simulink model "simulink_app"  (R2015a)
settings: Solver=ode2  SolverMode=SingleTasking  StartTime=0.0  StopTime=inf  FixedStep=T_ctrl  RelTol=1e-3
undefined symbols (not defined in the file): A_l_max_x, A_l_max_y, A_z_max, B_hover_4dof, CG_0, epsilon, eta_23, g, h, h_M, Hover_eta_23, Hover_throtle_1, Hover_throtle_23, I_BAC_0, Ix, Iy, Iz, l, l_arm, m, m_0, m_M, Rotation_sign, T_ctrl, throtle_1, throtle_23, v_i0
libraries: XXCopter_Control x52, simulink x11, XXCopter x1
(part 3 of 4)

== system simulink_app/Flight mode manager and commands generator/Commands generator/Take off ==
  Init comands : Inport
  Gains : Inport  Port=2
  Left_up : Inport  Port=3
  Left_side : Inport  Port=4
  Right_up : Inport  Port=5
  Right_side : Inport  Port=6
  GCS_comm : Inport  Port=7
  Enable : EnablePort  StatesWhenEnabling=reset  ShowOutputPort=on
  Bus Selector : BusSelector  OutputSignals=K_alt
  Bus Selector1 : BusSelector  OutputSignals=Alt_sp
  Bus Selector2 : BusSelector  OutputSignals=Alt_com
  Divide : Product  Inputs=**
  GCS params safemode : XXCopter_Control/GCS params safemode
  Ground{,1..4} (5 alike) : Ground
  Mux : Mux  Inputs=[2,1]
  Mux1 : Mux  Inputs=[2,1]
  Mux2 : Mux  Inputs=3
  Sum : Sum  Inputs=|++
  Sum1 : Sum  Inputs=|++
  Terminator : Terminator
  Terminator1 : Terminator
  Terminator2 : Terminator
  Unary Minus : UnaryMinus
  Pos_ref(m) : Outport
  Vel_ref_yaw(mps) : Outport  Port=2
  Att_ref(rad) : Outport  Port=3
  omega_b_ref : Outport  Port=4
  wires:
  Mux1/1 -> Vel_ref_yaw(mps)/1
  Mux/1 -> Pos_ref(m)/1
  Mux2/1 -> Att_ref(rad)/1
  Gains/1 -> Bus Selector/1
  Init comands/1 -> Bus Selector1/1
  Unary Minus/1 -> Mux/2
  GCS_comm/1 -> Bus Selector2/1
  Bus Selector1/1 -> Sum/1  "<Alt_sp>"
  Bus Selector/1 -> Divide/1  "<K_alt>"
  Left_up/1 -> Divide/2
  Divide/1 -> Sum/2
  Sum/1 -> Sum1/1
  GCS params safemode/1 -> Sum1/2
  Sum1/1 -> Unary Minus/1
  Right_up/1 -> Terminator/1
  Left_side/1 -> Terminator1/1
  Right_side/1 -> Terminator2/1
  Ground/1 -> omega_b_ref/1
  Ground1/1 -> Mux2/3, Mux2/2, Mux2/1
  Ground2/1 -> Mux1/1
  Ground3/1 -> Mux1/2
  Ground4/1 -> Mux/1
  Enable/1 -> GCS params safemode/1
  Bus Selector2/1 -> GCS params safemode/2  "<Alt_com>"

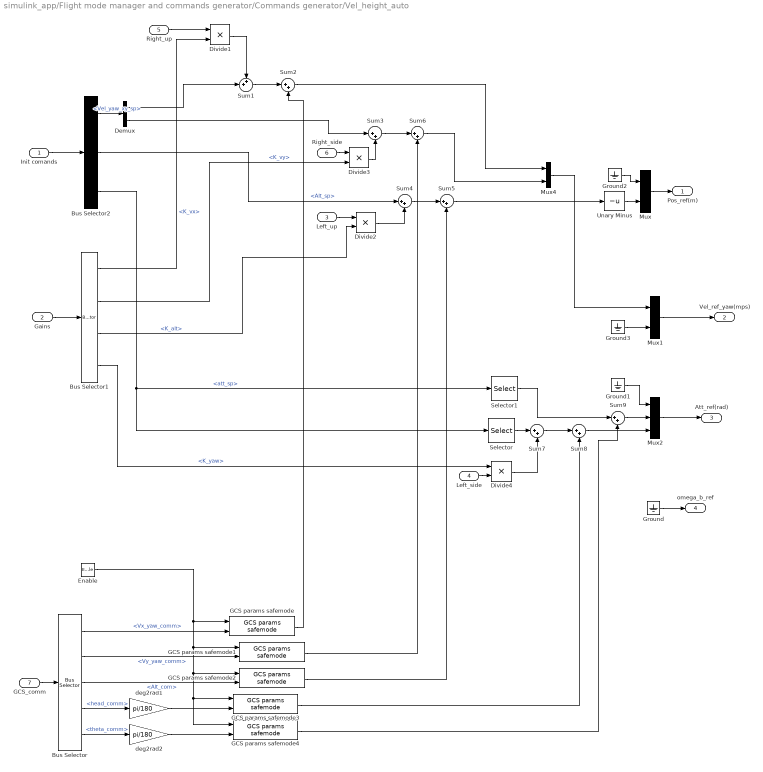
== system simulink_app/Flight mode manager and commands generator/Commands generator/Vel_height_auto ==
  Init comands : Inport
  Gains : Inport  Port=2
  Left_up : Inport  Port=3
  Left_side : Inport  Port=4
  Right_up : Inport  Port=5
  Right_side : Inport  Port=6
  GCS_comm : Inport  Port=7
  Enable : EnablePort  StatesWhenEnabling=reset  ShowOutputPort=on
  Bus Selector : BusSelector  OutputSignals=Vx_yaw_comm,Vy_yaw_comm,Alt_com,head_comm,theta_comm
  Bus Selector1 : BusSelector  OutputSignals=K_vx,K_vy,K_alt,K_yaw
  Bus Selector2 : BusSelector  OutputSignals=Vel_yaw_xy_sp,Alt_sp,att_sp
  Demux : Demux  Outputs=2
  Divide{1..4} (4 alike) : Product  Inputs=**
  GCS params safemode{,1..4} (5 alike) : XXCopter_Control/GCS params safemode
  Ground{,1..3} (4 alike) : Ground
  Mux : Mux  Inputs=[2,1]
  Mux1 : Mux  Inputs=[2,1]
  Mux2 : Mux  Inputs=3
  Mux4 : Mux  Inputs=2
  Selector : Selector  InputPortWidth=3  Indices=3
  Selector1 : Selector  InputPortWidth=3  Indices=2
  Sum1 : Sum  Inputs=++|
  Sum{2..9} (8 alike) : Sum  Inputs=|++
  Unary Minus : UnaryMinus
  deg2rad1 : Gain  Gain=pi/180
  deg2rad2 : Gain  Gain=pi/180
  Pos_ref(m) : Outport
  Vel_ref_yaw(mps) : Outport  Port=2
  Att_ref(rad) : Outport  Port=3
  omega_b_ref : Outport  Port=4
  wires:
  Mux1/1 -> Vel_ref_yaw(mps)/1
  Mux2/1 -> Att_ref(rad)/1
  Unary Minus/1 -> Mux/2
  Ground1/1 -> Mux2/1
  Mux4/1 -> Mux1/1
  Ground3/1 -> Mux1/2
  Ground/1 -> omega_b_ref/1
  Mux/1 -> Pos_ref(m)/1
  Gains/1 -> Bus Selector1/1
  Init comands/1 -> Bus Selector2/1
  GCS_comm/1 -> Bus Selector/1
  Sum4/1 -> Sum5/1
  Divide2/1 -> Sum4/2
  Bus Selector2/2 -> Sum4/1  "<Alt_sp>"
  Bus Selector2/1 -> Demux/1  "<Vel_yaw_xy_sp>"
  Sum1/1 -> Sum2/1
  Demux/1 -> Sum1/2
  Right_up/1 -> Divide1/1
  Divide1/1 -> Sum1/1
  Bus Selector1/1 -> Divide1/2  "<K_vx>"
  Bus Selector/1 -> GCS params safemode/2  "<Vx_yaw_comm>"
  GCS params safemode/1 -> Sum2/2
  Bus Selector/2 -> GCS params safemode1/2  "<Vy_yaw_comm>"
  Bus Selector/3 -> GCS params safemode2/2  "<Alt_com>"
  Bus Selector/4 -> deg2rad1/1  "<head_comm>"
  Bus Selector/5 -> deg2rad2/1  "<theta_comm>"
  GCS params safemode2/1 -> Sum5/2
  Sum5/1 -> Unary Minus/1
  Bus Selector1/3 -> Divide2/2  "<K_alt>"
  Left_up/1 -> Divide2/1
  Sum3/1 -> Sum6/1
  Divide3/1 -> Sum3/2
  Right_side/1 -> Divide3/1
  Bus Selector1/2 -> Divide3/2  "<K_vy>"
  Demux/2 -> Sum3/1
  Sum2/1 -> Mux4/1
  Sum6/1 -> Mux4/2
  GCS params safemode1/1 -> Sum6/2
  Sum7/1 -> Sum8/1
  Selector/1 -> Sum7/1
  Left_side/1 -> Divide4/2
  Bus Selector2/3 -> Selector/1, Selector1/1  "<att_sp>"
  Bus Selector1/4 -> Divide4/1  "<K_yaw>"
  Sum8/1 -> Mux2/3
  Selector1/1 -> Sum9/1
  Sum9/1 -> Mux2/2
  Divide4/1 -> Sum7/2
  GCS params safemode3/1 -> Sum8/2
  GCS params safemode4/1 -> Sum9/2
  Ground2/1 -> Mux/1
  deg2rad1/1 -> GCS params safemode3/2
  deg2rad2/1 -> GCS params safemode4/2
  Enable/1 -> GCS params safemode4/1, GCS params safemode3/1, GCS params safemode2/1, GCS params safemode1/1, GCS params safemode/1

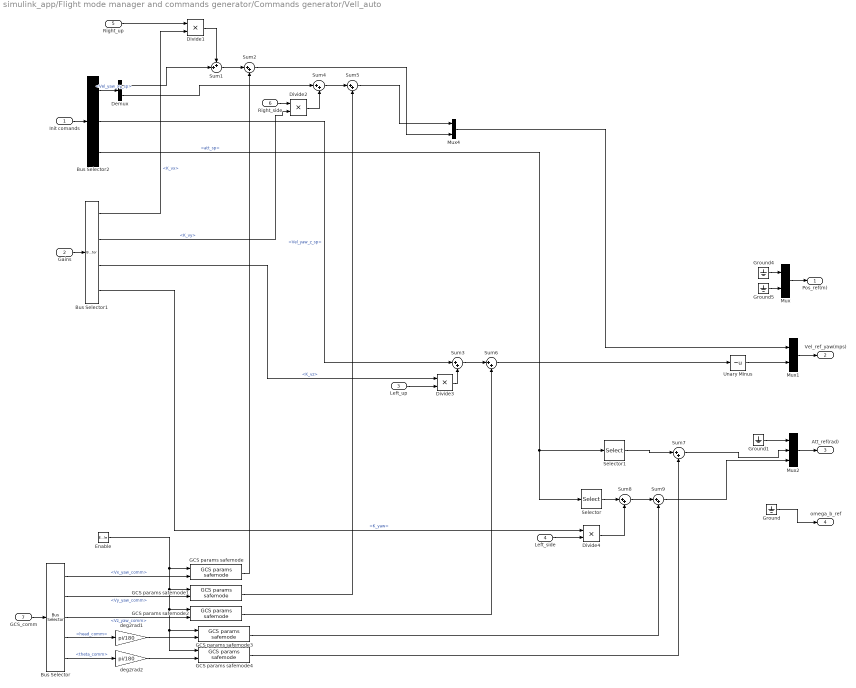
== system simulink_app/Flight mode manager and commands generator/Commands generator/Vell_auto ==
  Init comands : Inport
  Gains : Inport  Port=2
  Left_up : Inport  Port=3
  Left_side : Inport  Port=4
  Right_up : Inport  Port=5
  Right_side : Inport  Port=6
  GCS_comm : Inport  Port=7
  Enable : EnablePort  StatesWhenEnabling=reset  ShowOutputPort=on
  Bus Selector : BusSelector  OutputSignals=Vx_yaw_comm,Vy_yaw_comm,Vz_yaw_comm,head_comm,theta_comm
  Bus Selector1 : BusSelector  OutputSignals=K_vx,K_vy,K_vz,K_yaw
  Bus Selector2 : BusSelector  OutputSignals=Vel_yaw_xy_sp,Vel_yaw_z_sp,att_sp
  Demux : Demux  Outputs=2
  Divide{1..4} (4 alike) : Product  Inputs=**
  GCS params safemode{,1..4} (5 alike) : XXCopter_Control/GCS params safemode
  Ground{,1,4..5} (4 alike) : Ground
  Mux : Mux  Inputs=[2,1]
  Mux1 : Mux  Inputs=[2,1]
  Mux2 : Mux  Inputs=3
  Mux4 : Mux  Inputs=2
  Selector : Selector  InputPortWidth=3  Indices=3
  Selector1 : Selector  InputPortWidth=3  Indices=2
  Sum1 : Sum  Inputs=++|
  Sum{2..9} (8 alike) : Sum  Inputs=|++
  Unary Minus : UnaryMinus
  deg2rad1 : Gain  Gain=pi/180
  deg2rad2 : Gain  Gain=pi/180
  Pos_ref(m) : Outport
  Vel_ref_yaw(mps) : Outport  Port=2
  Att_ref(rad) : Outport  Port=3
  omega_b_ref : Outport  Port=4
  wires:
  Mux1/1 -> Vel_ref_yaw(mps)/1
  Mux2/1 -> Att_ref(rad)/1
  Ground1/1 -> Mux2/1
  Mux/1 -> Pos_ref(m)/1
  GCS_comm/1 -> Bus Selector/1
  Bus Selector/1 -> GCS params safemode/2  "<Vx_yaw_comm>"
  Bus Selector/2 -> GCS params safemode1/2  "<Vy_yaw_comm>"
  Bus Selector/3 -> GCS params safemode2/2  "<Vz_yaw_comm>"
  Bus Selector/4 -> deg2rad1/1  "<head_comm>"
  Bus Selector/5 -> deg2rad2/1  "<theta_comm>"
  Bus Selector2/1 -> Demux/1  "<Vel_yaw_xy_sp>"
  Gains/1 -> Bus Selector1/1
  Init comands/1 -> Bus Selector2/1
  Sum3/1 -> Sum6/1
  Divide3/1 -> Sum3/2
  Left_up/1 -> Divide3/2
  Bus Selector1/3 -> Divide3/1  "<K_vz>"
  Ground5/1 -> Mux/2
  Ground4/1 -> Mux/1
  Bus Selector2/2 -> Sum3/1  "<Vel_yaw_z_sp>"
  GCS params safemode2/1 -> Sum6/2
  Unary Minus/1 -> Mux1/2
  Sum6/1 -> Unary Minus/1
  Sum1/1 -> Sum2/1
  Demux/1 -> Sum1/2
  Right_up/1 -> Divide1/1
  Divide1/1 -> Sum1/1
  Bus Selector1/1 -> Divide1/2  "<K_vx>"
  GCS params safemode/1 -> Sum2/2
  Sum4/1 -> Sum5/1
  Demux/2 -> Sum4/1
  Sum2/1 -> Mux4/2
  GCS params safemode1/1 -> Sum5/2
  Sum5/1 -> Mux4/1
  Divide2/1 -> Sum4/2
  Bus Selector1/2 -> Divide2/2  "<K_vy>"
  Right_side/1 -> Divide2/1
  Mux4/1 -> Mux1/1
  Sum8/1 -> Sum9/1
  Selector/1 -> Sum8/1
  Bus Selector2/3 -> Selector1/1, Selector/1  "<att_sp>"
  Left_side/1 -> Divide4/2
  Divide4/1 -> Sum8/2
  Sum9/1 -> Mux2/3
  GCS params safemode3/1 -> Sum9/2
  Bus Selector1/4 -> Divide4/1  "<K_yaw>"
  Sum7/1 -> Mux2/2
  GCS params safemode4/1 -> Sum7/2
  Selector1/1 -> Sum7/1
  deg2rad1/1 -> GCS params safemode3/2
  deg2rad2/1 -> GCS params safemode4/2
  Enable/1 -> GCS params safemode4/1, GCS params safemode3/1, GCS params safemode2/1, GCS params safemode1/1, GCS params safemode/1
  Ground/1 -> omega_b_ref/1

== system simulink_app/Flight mode manager and commands generator/Commands generator/commnads_gen_logic ==
  flight_mode : Inport
  All_meas : Inport  Port=2
  Enable : EnablePort  StatesWhenEnabling=reset
  Bus Creator : BusCreator  Inputs=12  OutDataTypeStr=Bus: manual_gains
  Bus Creator1 : BusCreator  Inputs=6  OutDataTypeStr=Bus: commander_sp
  Bus Selector1 : BusSelector  OutputSignals=Meas.Pos_meas_m,Params.V_yaw,Meas.Eulr_meas_rad
  Signal Conversion : SignalConversion
  Signal Conversion1 : SignalConversion
  commands_generator : MATLAB Function  TreatAsAtomicUnit=on
  set_points : Outport
  gains : Outport  Port=2
  wires:
  All_meas/1 -> Bus Selector1/1
  Bus Selector1/1 -> commands_generator/2(Xe)  "<Pos_meas_m>"
  Bus Selector1/2 -> commands_generator/3(V_yaw)  "<V_yaw>"
  Bus Selector1/3 -> commands_generator/4(Euler)  "<Eulr_meas_rad>"
  commands_generator/1(Loc_XY_sp) -> Bus Creator1/1  "Loc_XY_sp"
  commands_generator/2(Alt_sp) -> Bus Creator1/2  "Alt_sp"
  commands_generator/3(Vel_yaw_xy_sp) -> Bus Creator1/3  "Vel_yaw_xy_sp"
  commands_generator/4(Vel_yaw_z_sp) -> Bus Creator1/4  "Vel_yaw_z_sp"
  commands_generator/5(att_sp) -> Bus Creator1/5  "att_sp"
  commands_generator/16(K_p) -> Bus Creator/10  "K_p"
  commands_generator/17(K_q) -> Bus Creator/11  "K_q"
  commands_generator/18(K_r) -> Bus Creator/12  "K_r"
  Bus Creator/1 -> Signal Conversion1/1  "manual_gains"
  flight_mode/1 -> commands_generator/1(flight_mode)
  commands_generator/6(omega_b_sp) -> Bus Creator1/6  "omega_b_sp"
  commands_generator/7(K_alt) -> Bus Creator/1  "K_alt"
  commands_generator/8(K_x) -> Bus Creator/2  "K_x"
  commands_generator/9(K_y) -> Bus Creator/3  "K_y"
  commands_generator/15(K_yaw) -> Bus Creator/9  "K_yaw"
  commands_generator/10(K_vx) -> Bus Creator/4  "K_vx"
  commands_generator/11(K_vy) -> Bus Creator/5  "K_vy"
  commands_generator/12(K_vz) -> Bus Creator/6  "K_vz"
  commands_generator/13(K_phi) -> Bus Creator/7  "K_phi"
  commands_generator/14(K_theta) -> Bus Creator/8  "K_theta"
  Bus Creator1/1 -> Signal Conversion/1  "commander_sp"
  Signal Conversion/1 -> set_points/1
  Signal Conversion1/1 -> gains/1

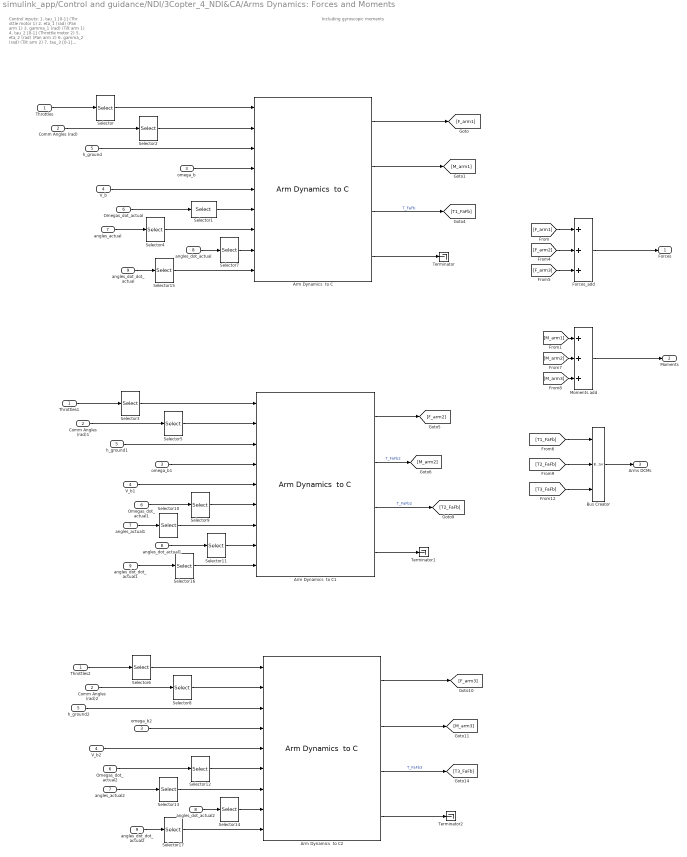
== system simulink_app/Control and guidance/NDI/3Copter_4_NDI&CA/Arms Dynamics: Forces and Moments ==
  note: Including gyroscopic moments
  note: Control inputs:
      | 1. tau_1 [0-1] (Thr ottle motor 1)
      | 2. eta_1 (rad)  (Pan arm 1)
      | 3. gamma_1 (rad)  (Tilt arm 1)
      |
      | 4. tau_2 [0-1] (Throttle motor 2)
      | 5. eta_2 (rad)  (Pan arm 2)
      | 6. gamma_2 (rad)  (Tilt arm 2)
      |
      | 7. tau_3 [0-1] (Throttle motor 3)
      | 8. eta_3 (rad)  (Pan arm  3)
      | 9. gamma_3 (rad)  (Tilt arm 3)
  Throttles : Inport
  Comm Angles (rad) : Inport  Port=2
  omega_b : Inport  Port=3
  V_b : Inport  Port=4
  h_ground : Inport  Port=5
  Omegas_dot_actual : Inport  Port=6
  angles_actual : Inport  Port=7
  angles_dot_actual : Inport  Port=8
  angles_dot_dot_actual : Inport  Port=9
  Arm Dynamics  to C : XXCopter_Control/Arm Dynamics  to C  Rot_sign=Rotation_sign(1)  arm_hub_pos=l*[1;0;0]  Arm_axis=[l_arm;0;0]  arm_num=1  eta_dir=[1;0;0]  gamma_dir=[0;1;0]  J_T=J_T  J_FA=J_FA  h=h  switch_val=direct_feedforward  omega_n=30  xi=1.4  eta_inf_lim=deg2rad(-180)  eta_sup_lim=deg2rad(180)  gamma_inf_lim=deg2rad(-90)  gamma_sup_lim=deg2rad(15)
  Arm Dynamics  to C1 : XXCopter_Control/Arm Dynamics  to C  Rot_sign=Rotation_sign(2)  arm_hub_pos=l*[-1/2;sqrt(3)/2;0]  Arm_axis=[0;l_arm;0]  arm_num=2  eta_dir=[0;1;0]  gamma_dir=[1;0;0]  J_T=J_T  J_FA=J_FA  h=h  switch_val=direct_feedforward  omega_n=30  xi=1.4  eta_inf_lim=deg2rad(-180)  eta_sup_lim=deg2rad(180)  gamma_inf_lim=deg2rad(-15)  gamma_sup_lim=deg2rad(90)
  Arm Dynamics  to C2 : XXCopter_Control/Arm Dynamics  to C  Rot_sign=Rotation_sign(3)  arm_hub_pos=l*[-1/2;-sqrt(3)/2;0]  Arm_axis=[0;-l_arm;0]  arm_num=3  eta_dir=[0;1;0]  gamma_dir=[1;0;0]  J_T=J_T  J_FA=J_FA  h=h  switch_val=direct_feedforward  omega_n=30  xi=1.4  eta_inf_lim=deg2rad(-180)  eta_sup_lim=deg2rad(180)  gamma_inf_lim=deg2rad(-90)  gamma_sup_lim=deg2rad(15)
  Bus Creator : BusCreator  Inputs=3
  Comm Angles (rad)1 : InportShadow  Port=2
  Comm Angles (rad)2 : InportShadow  Port=2
  Forces_add : Sum  Inputs=+++
  Moments add : Sum  Inputs=+++
  Omegas_dot_actual1 : InportShadow  Port=6
  Omegas_dot_actual2 : InportShadow  Port=6
  Selector : Selector  IndexMode=Zero-based  InputPortWidth=3  Indices=0
  Selector1 : Selector  IndexMode=Zero-based  InputPortWidth=3  Indices=0
  Selector{5,10..11,16} (4 alike) : Selector  IndexMode=Zero-based  InputPortWidth=6  Indices=[2,3]
  Selector12 : Selector  IndexMode=Zero-based  InputPortWidth=3  Indices=2
  Selector{8,13..14,17} (4 alike) : Selector  IndexMode=Zero-based  InputPortWidth=6  Indices=[4,5]
  Selector{2,4,7,15} (4 alike) : Selector  IndexMode=Zero-based  InputPortWidth=6  Indices=[0,1]
  Selector3 : Selector  IndexMode=Zero-based  InputPortWidth=3
  Selector6 : Selector  IndexMode=Zero-based  InputPortWidth=3  Indices=2
  Selector9 : Selector  IndexMode=Zero-based  InputPortWidth=3
  Terminator : Terminator
  Terminator1 : Terminator
  Terminator2 : Terminator
  Throttles1 : InportShadow
  Throttles2 : InportShadow
  V_b1 : InportShadow  Port=4
  V_b2 : InportShadow  Port=4
  angles_actual1 : InportShadow  Port=7
  angles_actual2 : InportShadow  Port=7
  angles_dot_actual1 : InportShadow  Port=8
  angles_dot_actual2 : InportShadow  Port=8
  angles_dot_dot_actual1 : InportShadow  Port=9
  angles_dot_dot_actual2 : InportShadow  Port=9
  h_ground1 : InportShadow  Port=5
  h_ground2 : InportShadow  Port=5
  omega_b1 : InportShadow  Port=3
  omega_b2 : InportShadow  Port=3
  Forces : Outport
  Moments : Outport  Port=2
  Arms DCMs : Outport  Port=3
  wires:
  Selector14/1 -> Arm Dynamics  to C2/8
  angles_actual2/1 -> Selector13/1
  angles_dot_actual2/1 -> Selector14/1
  Selector13/1 -> Arm Dynamics  to C2/7
  Selector12/1 -> Arm Dynamics  to C2/6
  Omegas_dot_actual2/1 -> Selector12/1
  Selector11/1 -> Arm Dynamics  to C1/8
  angles_actual1/1 -> Selector10/1
  angles_dot_actual1/1 -> Selector11/1
  Selector10/1 -> Arm Dynamics  to C1/7
  Selector9/1 -> Arm Dynamics  to C1/6
  Omegas_dot_actual1/1 -> Selector9/1
  Selector7/1 -> Arm Dynamics  to C/8
  angles_dot_actual/1 -> Selector7/1
  Selector4/1 -> Arm Dynamics  to C/7
  angles_actual/1 -> Selector4/1
  Selector1/1 -> Arm Dynamics  to C/6
  Omegas_dot_actual/1 -> Selector1/1
  [T3_FaFb] -> Bus Creator/3
  [T2_FaFb] -> Bus Creator/2
  [T1_FaFb] -> Bus Creator/1
  Bus Creator/1 -> Arms DCMs/1
  Arm Dynamics  to C1/2 -> [M_arm2]  "T_FaFb2"
  Arm Dynamics  to C1/1 -> [F_arm2]
  Arm Dynamics  to C2/4 -> Terminator2/1
  Arm Dynamics  to C1/4 -> Terminator1/1
  Arm Dynamics  to C/4 -> Terminator/1
  Arm Dynamics  to C2/3 -> [T3_FaFb]  "T_FaFb3"
  Comm Angles (rad)2/1 -> Selector8/1
  Selector8/1 -> Arm Dynamics  to C2/2
  omega_b2/1 -> Arm Dynamics  to C2/4
  Arm Dynamics  to C2/2 -> [M_arm3]
  Arm Dynamics  to C2/1 -> [F_arm3]
  h_ground2/1 -> Arm Dynamics  to C2/3
  V_b2/1 -> Arm Dynamics  to C2/5
  Selector6/1 -> Arm Dynamics  to C2/1
  Throttles2/1 -> Selector6/1
  Arm Dynamics  to C1/3 -> [T2_FaFb]  "T_FaFb2"
  Comm Angles (rad)1/1 -> Selector5/1
  Selector5/1 -> Arm Dynamics  to C1/2
  omega_b1/1 -> Arm Dynamics  to C1/4
  h_ground1/1 -> Arm Dynamics  to C1/3
  V_b1/1 -> Arm Dynamics  to C1/5
  Selector3/1 -> Arm Dynamics  to C1/1
  Throttles1/1 -> Selector3/1
  Arm Dynamics  to C/3 -> [T1_FaFb]  "T_FaFb"
  Comm Angles (rad)/1 -> Selector2/1
  Selector2/1 -> Arm Dynamics  to C/2
  [M_arm2] -> Moments add/2
  [M_arm3] -> Moments add/3
  [F_arm3] -> Forces_add/3
  [F_arm2] -> Forces_add/2
  omega_b/1 -> Arm Dynamics  to C/4
  [M_arm1] -> Moments add/1
  [F_arm1] -> Forces_add/1
  Arm Dynamics  to C/2 -> [M_arm1]
  Arm Dynamics  to C/1 -> [F_arm1]
  h_ground/1 -> Arm Dynamics  to C/3
  Moments add/1 -> Moments/1
  Forces_add/1 -> Forces/1
  V_b/1 -> Arm Dynamics  to C/5
  Selector/1 -> Arm Dynamics  to C/1
  Throttles/1 -> Selector/1
  angles_dot_dot_actual/1 -> Selector15/1
  Selector15/1 -> Arm Dynamics  to C/9
  angles_dot_dot_actual1/1 -> Selector16/1
  Selector16/1 -> Arm Dynamics  to C1/9
  angles_dot_dot_actual2/1 -> Selector17/1
  Selector17/1 -> Arm Dynamics  to C2/9

== system simulink_app/Control and guidance/NDI/3Copter_4_NDI&CA/Gradient ==
  note: Control inputs:
      | 1. tau_1 [0-1] (Thr ottle motor 1)
      | 2. eta_1 (rad)  (Pan arm 1)
      | 3. gamma_1 (rad)  (Tilt arm 1)
      |
      | 4. tau_2 [0-1] (Throttle motor 2)
      | 5. eta_2 (rad)  (Pan arm 2)
      | 6. gamma_2 (rad)  (Tilt arm 2)
      |
      | 7. tau_3 [0-1] (Throttle motor 3)
      | 8. eta_3 (rad)  (Pan arm  3)
      | 9. gamma_3 (rad)  (Tilt arm 3)
  Curr_V : Inport  Partition=off
  "Control Inputs(rad) " : Inport  Port=2  Partition=on  PartitionDimension=1  PartitionWidth=9
  h : Inport  Port=3  Partition=off
  Vb : Inport  Port=4  Partition=off
  omega_b : Inport  Port=5  Partition=off
  Omegas_dot_actual : Inport  Port=6  Partition=off
  angles_actual : Inport  Port=7  Partition=off
  angles_dot_actual : Inport  Port=8  Partition=off
  angles_dot_dot_actual : Inport  Port=9  Partition=off
  F_g : Inport  Port=10  Partition=off
  M_g : Inport  Port=11  Partition=off
  Add : Sum
  Add1 : Sum
  Arms Dynamics: Forces and Moments : Subsystem  TreatAsAtomicUnit=on
  Equivalent Throttle : Product  Inputs=**
  For Each : ForEach  DisableCoverage=on  IndexMode=One-based
  Mux : Mux  Inputs=[3,3]
  Signal Specification : SignalSpecification  Dimensions=[6,1]
  Terminator : Terminator
  Throttles : Selector  IndexMode=Zero-based  InputPortWidth=9  Indices=[0,3,6]
  "angles " : Selector  IndexMode=Zero-based  InputPortWidth=9  Indices=[1,2,4,5,7,8]
  Forces_Moments : Outport  ConcatenationDimension=2
  wires:
  Signal Specification/1 -> Forces_Moments/1
  Mux/1 -> Signal Specification/1
  Add1/1 -> Mux/2
  Add/1 -> Mux/1
  M_g/1 -> Add1/2
  F_g/1 -> Add/2
  angles_dot_actual/1 -> Arms Dynamics: Forces and Moments/8(angles_dot_actual)
  Omegas_dot_actual/1 -> Arms Dynamics: Forces and Moments/6(Omegas_dot_actual)
  Curr_V/1 -> Equivalent Throttle/1
  Equivalent Throttle/1 -> Arms Dynamics: Forces and Moments/1(Throttles)
  "Control Inputs(rad) "/1 -> "angles "/1, Throttles/1
  Throttles/1 -> Equivalent Throttle/2
  Arms Dynamics: Forces and Moments/1(Forces) -> Add/1
  h/1 -> Arms Dynamics: Forces and Moments/5(h_ground)
  omega_b/1 -> Arms Dynamics: Forces and Moments/3(omega_b)
  angles_actual/1 -> Arms Dynamics: Forces and Moments/7(angles_actual)
  "angles "/1 -> Arms Dynamics: Forces and Moments/2(Comm Angles (rad))
  angles_dot_dot_actual/1 -> Arms Dynamics: Forces and Moments/9(angles_dot_dot_actual)
  Arms Dynamics: Forces and Moments/2(Moments) -> Add1/1
  Arms Dynamics: Forces and Moments/3(Arms DCMs) -> Terminator/1
  Vb/1 -> Arms Dynamics: Forces and Moments/4(V_b)

== system simulink_app/Control and guidance/NDI/3Copter_4_NDI&CA/Ground  model ==
  h : Inport
  m : Inport  Port=2
  q : Inport  Port=3
  Ground model logic and Forces and moments : MATLAB Function  TreatAsAtomicUnit=on
  arm_hub position 1 : Constant  Value=l*[1;0;0]
  arm_hub position 2 : Constant  Value=l*[-1/2;sqrt(3)/2;0]
  arm_hub position 3 : Constant  Value=l*[-1/2;-sqrt(3)/2;0]
  F_ground : Outport
  wires:
  h/1 -> Ground model logic and Forces and moments/1(h)
  m/1 -> Ground model logic and Forces and moments/2(mass)
  arm_hub position 1/1 -> Ground model logic and Forces and moments/4(Arm1)
  arm_hub position 2/1 -> Ground model logic and Forces and moments/5(Arm2)
  arm_hub position 3/1 -> Ground model logic and Forces and moments/6(Arm3)
  Ground model logic and Forces and moments/1(F_gr_b) -> F_ground/1
  q/1 -> Ground model logic and Forces and moments/3(q)

== system simulink_app/Control and guidance/NDI/3Copter_4_NDI&CA/Mass Properties ==
  Arms DCMs : Inport
  CG_0 : Inport  Port=2
  m_0 : Inport  Port=3
  m : Inport  Port=4
  m_M : Inport  Port=5
  I_BAC_0 : Inport  Port=6
  Arm Inertia : MATLAB Function  TreatAsAtomicUnit=on
  Bus Selector : BusSelector  OutputSignals=T_FaFb,T_FaFb2,T_FaFb3
  CG position : Sum
  Divide : Product  Inputs=*/
  Divide1 : Product  Inputs=**
  Divide2 : Product  Inputs=/*
  Divide3 : Product  Inputs=**
  Motors Pos sum : Sum  Inputs=+++
  Total I_BAC : Sum
  I_BAC : Outport
  CG : Outport  Port=2
  wires:
  Arm Inertia/2(r1_M) -> Motors Pos sum/3
  I_BAC_0/1 -> Total I_BAC/1
  Arm Inertia/1(I_M) -> Total I_BAC/2
  Arm Inertia/4(r3_M) -> Motors Pos sum/1
  Arm Inertia/3(r2_M) -> Motors Pos sum/2
  Divide3/1 -> CG position/2
  Divide2/1 -> Divide3/2
  Motors Pos sum/1 -> Divide3/1
  Divide1/1 -> CG position/1
  CG position/1 -> CG/1
  m_M/1 -> Divide2/2
  Divide/1 -> Divide1/2
  CG_0/1 -> Divide1/1
  m/1 -> Divide2/1, Divide/2
  m_0/1 -> Divide/1
  Total I_BAC/1 -> I_BAC/1
  Bus Selector/1 -> Arm Inertia/1(T1_FAFb)  "<T_FaFb>"
  Bus Selector/2 -> Arm Inertia/2(T2_FAFb)  "<T_FaFb2>"
  Bus Selector/3 -> Arm Inertia/3(T3_FAFb)  "<T_FaFb3>"
  Arms DCMs/1 -> Bus Selector/1

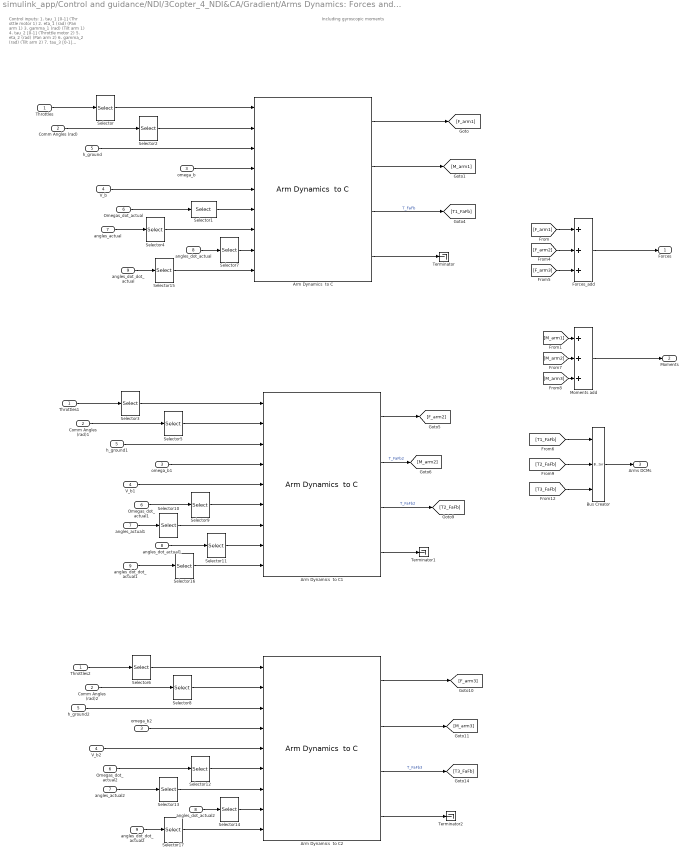
== system simulink_app/Control and guidance/NDI/3Copter_4_NDI&CA/Gradient/Arms Dynamics: Forces and Moments ==
  note: Including gyroscopic moments
  note: Control inputs:
      | 1. tau_1 [0-1] (Thr ottle motor 1)
      | 2. eta_1 (rad)  (Pan arm 1)
      | 3. gamma_1 (rad)  (Tilt arm 1)
      |
      | 4. tau_2 [0-1] (Throttle motor 2)
      | 5. eta_2 (rad)  (Pan arm 2)
      | 6. gamma_2 (rad)  (Tilt arm 2)
      |
      | 7. tau_3 [0-1] (Throttle motor 3)
      | 8. eta_3 (rad)  (Pan arm  3)
      | 9. gamma_3 (rad)  (Tilt arm 3)
  Throttles : Inport
  Comm Angles (rad) : Inport  Port=2
  omega_b : Inport  Port=3
  V_b : Inport  Port=4
  h_ground : Inport  Port=5
  Omegas_dot_actual : Inport  Port=6
  angles_actual : Inport  Port=7
  angles_dot_actual : Inport  Port=8
  angles_dot_dot_actual : Inport  Port=9
  Arm Dynamics  to C : XXCopter_Control/Arm Dynamics  to C  Rot_sign=Rotation_sign(1)  arm_hub_pos=l*[1;0;0]  Arm_axis=[l_arm;0;0]  arm_num=1  eta_dir=[1;0;0]  gamma_dir=[0;1;0]  J_T=J_T  J_FA=J_FA  h=h  switch_val=direct_feedforward  omega_n=30  xi=1.4  eta_inf_lim=deg2rad(-180)  eta_sup_lim=deg2rad(180)  gamma_inf_lim=deg2rad(-90)  gamma_sup_lim=deg2rad(15)
  Arm Dynamics  to C1 : XXCopter_Control/Arm Dynamics  to C  Rot_sign=Rotation_sign(2)  arm_hub_pos=l*[-1/2;sqrt(3)/2;0]  Arm_axis=[0;l_arm;0]  arm_num=2  eta_dir=[0;1;0]  gamma_dir=[1;0;0]  J_T=J_T  J_FA=J_FA  h=h  switch_val=direct_feedforward  omega_n=30  xi=1.4  eta_inf_lim=deg2rad(-180)  eta_sup_lim=deg2rad(180)  gamma_inf_lim=deg2rad(-15)  gamma_sup_lim=deg2rad(90)
  Arm Dynamics  to C2 : XXCopter_Control/Arm Dynamics  to C  Rot_sign=Rotation_sign(3)  arm_hub_pos=l*[-1/2;-sqrt(3)/2;0]  Arm_axis=[0;-l_arm;0]  arm_num=3  eta_dir=[0;1;0]  gamma_dir=[1;0;0]  J_T=J_T  J_FA=J_FA  h=h  switch_val=direct_feedforward  omega_n=30  xi=1.4  eta_inf_lim=deg2rad(-180)  eta_sup_lim=deg2rad(180)  gamma_inf_lim=deg2rad(-90)  gamma_sup_lim=deg2rad(15)
  Bus Creator : BusCreator  Inputs=3
  Comm Angles (rad)1 : InportShadow  Port=2
  Comm Angles (rad)2 : InportShadow  Port=2
  Forces_add : Sum  Inputs=+++
  Moments add : Sum  Inputs=+++
  Omegas_dot_actual1 : InportShadow  Port=6
  Omegas_dot_actual2 : InportShadow  Port=6
  Selector : Selector  IndexMode=Zero-based  InputPortWidth=3  Indices=0
  Selector1 : Selector  IndexMode=Zero-based  InputPortWidth=3  Indices=0
  Selector{5,10..11,16} (4 alike) : Selector  IndexMode=Zero-based  InputPortWidth=6  Indices=[2,3]
  Selector12 : Selector  IndexMode=Zero-based  InputPortWidth=3  Indices=2
  Selector{8,13..14,17} (4 alike) : Selector  IndexMode=Zero-based  InputPortWidth=6  Indices=[4,5]
  Selector{2,4,7,15} (4 alike) : Selector  IndexMode=Zero-based  InputPortWidth=6  Indices=[0,1]
  Selector3 : Selector  IndexMode=Zero-based  InputPortWidth=3
  Selector6 : Selector  IndexMode=Zero-based  InputPortWidth=3  Indices=2
  Selector9 : Selector  IndexMode=Zero-based  InputPortWidth=3
  Terminator : Terminator
  Terminator1 : Terminator
  Terminator2 : Terminator
  Throttles1 : InportShadow
  Throttles2 : InportShadow
  V_b1 : InportShadow  Port=4
  V_b2 : InportShadow  Port=4
  angles_actual1 : InportShadow  Port=7
  angles_actual2 : InportShadow  Port=7
  angles_dot_actual1 : InportShadow  Port=8
  angles_dot_actual2 : InportShadow  Port=8
  angles_dot_dot_actual1 : InportShadow  Port=9
  angles_dot_dot_actual2 : InportShadow  Port=9
  h_ground1 : InportShadow  Port=5
  h_ground2 : InportShadow  Port=5
  omega_b1 : InportShadow  Port=3
  omega_b2 : InportShadow  Port=3
  Forces : Outport
  Moments : Outport  Port=2
  Arms DCMs : Outport  Port=3
  wires:
  Selector14/1 -> Arm Dynamics  to C2/8
  angles_actual2/1 -> Selector13/1
  angles_dot_actual2/1 -> Selector14/1
  Selector13/1 -> Arm Dynamics  to C2/7
  Selector12/1 -> Arm Dynamics  to C2/6
  Omegas_dot_actual2/1 -> Selector12/1
  Selector11/1 -> Arm Dynamics  to C1/8
  angles_actual1/1 -> Selector10/1
  angles_dot_actual1/1 -> Selector11/1
  Selector10/1 -> Arm Dynamics  to C1/7
  Selector9/1 -> Arm Dynamics  to C1/6
  Omegas_dot_actual1/1 -> Selector9/1
  Selector7/1 -> Arm Dynamics  to C/8
  angles_dot_actual/1 -> Selector7/1
  Selector4/1 -> Arm Dynamics  to C/7
  angles_actual/1 -> Selector4/1
  Selector1/1 -> Arm Dynamics  to C/6
  Omegas_dot_actual/1 -> Selector1/1
  [T3_FaFb] -> Bus Creator/3
  [T2_FaFb] -> Bus Creator/2
  [T1_FaFb] -> Bus Creator/1
  Bus Creator/1 -> Arms DCMs/1
  Arm Dynamics  to C1/2 -> [M_arm2]  "T_FaFb2"
  Arm Dynamics  to C1/1 -> [F_arm2]
  Arm Dynamics  to C2/4 -> Terminator2/1
  Arm Dynamics  to C1/4 -> Terminator1/1
  Arm Dynamics  to C/4 -> Terminator/1
  Arm Dynamics  to C2/3 -> [T3_FaFb]  "T_FaFb3"
  Comm Angles (rad)2/1 -> Selector8/1
  Selector8/1 -> Arm Dynamics  to C2/2
  omega_b2/1 -> Arm Dynamics  to C2/4
  Arm Dynamics  to C2/2 -> [M_arm3]
  Arm Dynamics  to C2/1 -> [F_arm3]
  h_ground2/1 -> Arm Dynamics  to C2/3
  V_b2/1 -> Arm Dynamics  to C2/5
  Selector6/1 -> Arm Dynamics  to C2/1
  Throttles2/1 -> Selector6/1
  Arm Dynamics  to C1/3 -> [T2_FaFb]  "T_FaFb2"
  Comm Angles (rad)1/1 -> Selector5/1
  Selector5/1 -> Arm Dynamics  to C1/2
  omega_b1/1 -> Arm Dynamics  to C1/4
  h_ground1/1 -> Arm Dynamics  to C1/3
  V_b1/1 -> Arm Dynamics  to C1/5
  Selector3/1 -> Arm Dynamics  to C1/1
  Throttles1/1 -> Selector3/1
  Arm Dynamics  to C/3 -> [T1_FaFb]  "T_FaFb"
  Comm Angles (rad)/1 -> Selector2/1
  Selector2/1 -> Arm Dynamics  to C/2
  [M_arm2] -> Moments add/2
  [M_arm3] -> Moments add/3
  [F_arm3] -> Forces_add/3
  [F_arm2] -> Forces_add/2
  omega_b/1 -> Arm Dynamics  to C/4
  [M_arm1] -> Moments add/1
  [F_arm1] -> Forces_add/1
  Arm Dynamics  to C/2 -> [M_arm1]
  Arm Dynamics  to C/1 -> [F_arm1]
  h_ground/1 -> Arm Dynamics  to C/3
  Moments add/1 -> Moments/1
  Forces_add/1 -> Forces/1
  V_b/1 -> Arm Dynamics  to C/5
  Selector/1 -> Arm Dynamics  to C/1
  Throttles/1 -> Selector/1
  angles_dot_dot_actual/1 -> Selector15/1
  Selector15/1 -> Arm Dynamics  to C/9
  angles_dot_dot_actual1/1 -> Selector16/1
  Selector16/1 -> Arm Dynamics  to C1/9
  angles_dot_dot_actual2/1 -> Selector17/1
  Selector17/1 -> Arm Dynamics  to C2/9

== matlab function simulink_app/Control and guidance/Inner PI Controller Quaternions/Attitude Controller/Build Pseudo_theta ==
  data: q input size=[4,1]; Pseudo_theta output size=1
function Pseudo_theta    = F_Pseudo_theta( q)


%% Actitud en Angulos de Euler y sus derivadas.
Pseudo_theta=0;
Pseudo_theta = ( 2*q(2)*q(4)-2*q(1)*q(3) ); %  pseudo-theta




end

== matlab function simulink_app/Control and guidance/Inner PI Controller Quaternions/Attitude Controller/Build Pseudo_theta1 ==
  data: q input size=[4,1]; Pseudo_theta output size=1
function Pseudo_theta    = F_Pseudo_theta( q)


%% Actitud en Angulos de Euler y sus derivadas.
Pseudo_theta=0;
Pseudo_theta = ( 2*q(2)*q(4)-2*q(1)*q(3) ); %  pseudo-theta




end

== matlab function simulink_app/Control and guidance/Inner PI Controller Quaternions/Attitude Controller/Retrieve quaternion ==
  data: Pseudoeuler_dot input size=[3,1]; q input size=[4,1]; qdot output size=[4,1]
function qdot = quat_from_Pseudoeuler(Pseudoeuler_dot, q)


%%
A = [   2/(1+( (2*q(3)*q(4)+2*q(1)*q(2))/(2*q(1)^2+2*q(4)^2-1)  )^2)*[ -(2*q(1)^2*q(2)+ 4*q(1)*q(3)*q(4)-2*q(2)*q(4)^2+q(2))  ,  q(1)*(2*q(1)^2+2*q(4)^2-1)  ,  q(4)*(2*q(1)^2+2*q(4)^2-1)  ,  -(-2*q(1)^2*q(3) +4*q(1)*q(2)*q(4)+2*q(3)*q(4)^2+q(3) ) ].* 1/(2*q(1)^2+2*q(4)^2-1)^2;...
        2*[-q(3),q(4),-q(1),q(2)];...
        2/(1+( (2*q(2)*q(3)+2*q(1)*q(4))/(2*q(1)^2+2*q(2)^2-1)  )^2)*[  -(2*q(1)^2*q(4)+4*q(1)*q(2)*q(3)-2*q(2)^2*q(4)+q(4)  ) , 1/2*(q(3)*(4*q(1)^2-4*q(2)^2-2)-8*q(1)*q(2)*q(4) )  ,  q(2)*(2*q(1)^2+2*q(2)^2-1)  , q(1)*(2*q(1)^2+2*q(2)^2-1) ].*  1/(2*q(1)^2+2*q(2)^2-1)^2 ;...
        2*[q(1),q(2),q(3),q(4)]];

qdot = pinv(A)*[Pseudoeuler_dot;0];

end

== matlab function simulink_app/Control and guidance/Inner PI Controller Quaternions/Get Quaternion from des euler ==
  data: phi input size=1; q output size=[4,1]; theta input size=1; psi input size=1
function q =QuaternionfromEuler(phi,theta,psi)

q=[ cos(psi/2)*cos(theta/2)*cos(phi/2)+ sin(psi/2)*sin(theta/2)*sin(phi/2) ;
      cos(psi/2)*cos(theta/2)*sin(phi/2)- sin(psi/2)*sin(theta/2)*cos(phi/2) ;
       cos(psi/2)*sin(theta/2)*cos(phi/2)+ sin(psi/2)*cos(theta/2)*sin(phi/2)   ;
        sin(psi/2)*cos(theta/2)*cos(phi/2)- cos(psi/2)*sin(theta/2)*sin(phi/2)      ]; % Esto nos da q !!!
end

== matlab function simulink_app/Control and guidance/Inner PI Controller Quaternions/Limits in Ang accel/Limis eval ==
  data: Ang_Accel input size=[3,1]; Limit_up output size=[3,1]; euler_ang input size=[3,1]; Limit_down output size=[3,1]; l parameter size=1; m parameter size=1; g parameter size=1; A_l_max_x parameter size=1; Ix parameter size=1; Iy parameter size=1; Iz parameter size=1
function [Limit_up,Limit_down]= Max_ang_accels(Ang_Accel,euler_ang,l,m,g,A_l_max_x,Ix,Iy,Iz)

Limit_up=Ang_Accel;
Limit_down=Ang_Accel;

Limit_up(1) = max(   abs( (2*m*g/3*sqrt(3)/2*l  )/Ix*cos(euler_ang(1))   ), abs(  2/3*A_l_max_x*sqrt(3)/2*l/Ix*sin(euler_ang(2)) ) )* 0.5 ;
Limit_down(1) = -Limit_up(1) ;

Limit_up(2) = max(  (l*m*g*2/3-l/2*m*g/3)/Iy*cos(euler_ang(2)) , (2*l*A_l_max_x)/Iy*sin(euler_ang(2)) )* 0.5 ;
Limit_down(2) = - max( (l/2*m*g)/Iy*cos(euler_ang(2))  , (2*l*A_l_max_x)/Iy*sin(euler_ang(2)) )* 0.5 ;


Limit_up(3) = max(  abs(  A_l_max_x*l/Iz*cos(euler_ang(1))*cos(euler_ang(2)) ) , abs(  (2*m*g/3*sqrt(3)/2*l  )/Iz*sin(euler_ang(2)) )  )* 0.5 ;
Limit_down(3) = -Limit_up(1) ;

== matlab function simulink_app/Control and guidance/Inner PI Controller Quaternions/MATLAB Function ==
  data: omega_b input size=[3,1]; Euler_dot output size=[3,1]; Euler input size=[3,1]
function Euler_dot = omega2Euler_dot(omega_b,Euler)

phi = Euler(1);
theta = Euler(2);
psi = Euler(3);


A = [1          0               -sin(theta)         ;
     0          cos(phi)        sin(phi)*cos(theta) ;
     0          -sin(phi)       cos(phi)*cos(theta)];

Euler_dot = A'*omega_b ;

== matlab function simulink_app/Control and guidance/Inner PI Controller Quaternions/Quaternion_dot ==
  data: omega_b output size=[3,1]; q_dot input size=[4,1]; q input size=[4,1]
function omega_b = Quaternion_dot(q_dot,q)

% omega_b = 2.q'*q_dot
out = 2*HamiltonProduct([q(1);- q(2:4)],q_dot);

omega_b = out(2:4);


function Product= HamiltonProduct( a,b )

Product=[ a(1)*b(1)-a(2)*b(2)-a(3)*b(3)-a(4)*b(4) ; a(1)*b(2)+a(2)*b(1)+a(3)*b(4)-a(4)*b(3)  ; a(1)*b(3)-a(2)*b(4)+a(3)*b(1)+a(4)*b(2)  ; a(1)*b(4)+a(2)*b(3)-a(3)*b(2)+a(4)*b(1) ];

== matlab function simulink_app/Control and guidance/NDI/3Copter_4_NDI&CA/Get gradient ==
  data: epsilon input size=1; CA_Grad output size=[6,9]; Perturb_evaluations input size=[6,18]
function CA_Grad  = Get_gradient(epsilon,Perturb_evaluations)

CA_Grad = zeros(6,9);

for i=1:9
    CA_Grad(:,i)= ( Perturb_evaluations(:,2*i)-Perturb_evaluations(:,2*i-1)  )./(epsilon);
end

%% 4 DOF
% CA_Grad(:,3)=zeros(6,1);
% CA_Grad(:,5:6)=zeros(6,2);
% CA_Grad(:,8:9)=zeros(6,2);
% 

%% Just diff throtle
% CA_Grad(3:5,2:3)=zeros(3,2);
% CA_Grad(3:5,5:6)=zeros(3,2);
% CA_Grad(3:5,8:9)=zeros(3,2);


end

== matlab function simulink_app/Control and guidance/NDI/3Copter_4_NDI&CA/Ground  model/Ground model logic and Forces and moments ==
  data: h input; F_gr_b output; mass input; q input; g parameter; Arm1 input; Arm2 input; Arm3 input
function F_gr_b    = Gorund_Forces_and_Mom( h,mass, q,g, Arm1,Arm2,Arm3)

F_gr_b=zeros(3,1);
min_h=0;

% Arm 1
Prod=HamiltonProduct([q(1);q(2);q(3);q(4)],HamiltonProduct([0;Arm1],[q(1);-q(2);-q(3);-q(4)]) ); % q . Arm .q*: From body to earth axes
h_arm1 = h + Prod(4);
% Arm 2
Prod=HamiltonProduct([q(1);q(2);q(3);q(4)],HamiltonProduct([0;Arm2],[q(1);-q(2);-q(3);-q(4)]) ); % q . Arm .q*: From body to earth axes
h_arm2 = h + Prod(4);
% Arm 3
Prod=HamiltonProduct([q(1);q(2);q(3);q(4)],HamiltonProduct([0;Arm3],[q(1);-q(2);-q(3);-q(4)]) ); % q . Arm .q*: From body to earth axes
h_arm3 = h + Prod(4);


min_h = max([h,h_arm1,h_arm2,h_arm3]);
if min_h >=-0.05 
    Prod=HamiltonProduct([q(1);-q(2);-q(3);-q(4)],HamiltonProduct([0;0;0;-mass*g],[q(1);q(2);q(3);q(4)]) ); % q* . g .q: From earth to Body axes
    F_gr_b= Prod(2:4);    
else
    F_gr_b=zeros(3,1);

end

function Product= HamiltonProduct( a,b )

Product=[ a(1)*b(1)-a(2)*b(2)-a(3)*b(3)-a(4)*b(4) ; a(1)*b(2)+a(2)*b(1)+a(3)*b(4)-a(4)*b(3)  ; a(1)*b(3)-a(2)*b(4)+a(3)*b(1)+a(4)*b(2)  ; a(1)*b(4)+a(2)*b(3)-a(3)*b(2)+a(4)*b(1) ];

== matlab function simulink_app/Control and guidance/NDI/3Copter_4_NDI&CA/Mass Properties/Arm Inertia ==
  data: T1_FAFb input; T2_FAFb input; T3_FAFb input; I_M output; l parameter; h_M parameter; m_M parameter; r1_M output; r2_M output; r3_M output
function [I_M,r1_M,r2_M,r3_M]  = Motor_steiner(T1_FAFb,T2_FAFb,T3_FAFb, l, h_M, m_M)


r1_M=[l;0;0]+T1_FAFb*[0;0;-h_M];
r2_M=[-1/2*l;sqrt(3)/2*l;0]+T2_FAFb*[0;0;-h_M];
r3_M=[-1/2*l;-sqrt(3)/2*l;0]+T3_FAFb*[0;0;-h_M];


I_M1 = m_M*[ r1_M(2)^2+r1_M(3)^2,r1_M(1)*r1_M(2),r1_M(1)*r1_M(3);...
            r1_M(1)*r1_M(2), r1_M(1)^2+r1_M(3)^2, r1_M(2)*r1_M(3);...
            r1_M(1)*r1_M(3),r1_M(2)*r1_M(3), r1_M(1)^2+r1_M(2)^2];
I_M2 = m_M*[ r2_M(2)^2+r2_M(3)^2,r2_M(1)*r2_M(2),r2_M(1)*r2_M(3);...
            r2_M(1)*r2_M(2), r2_M(1)^2+r2_M(3)^2, r2_M(2)*r2_M(3);...
            r2_M(1)*r2_M(3),r2_M(2)*r2_M(3), r2_M(1)^2+r2_M(2)^2];
I_M3 = m_M*[ r3_M(2)^2+r3_M(3)^2,r3_M(1)*r3_M(2),r3_M(1)*r3_M(3);...
            r3_M(1)*r3_M(2), r3_M(1)^2+r3_M(3)^2, r3_M(2)*r3_M(3);...
            r3_M(1)*r3_M(3),r3_M(2)*r3_M(3), r3_M(1)^2+r3_M(2)^2];

I_M = I_M1+I_M2+I_M3;

== matlab function simulink_app/Control and guidance/NDI/3Copter_4_NDI&CA/Perturbations ==
  data: epsilon input size=1; Ctrl_input input size=[9,1]; Pert_Ctrl output size=162
function Pert_Ctrl  = Perturbate_input(epsilon, Ctrl_input)
% The control input has a dimension of 9
% The gradient is computed with 2 evaluations, so the output vector has
% 2*9*9 variables

Pert_Ctrl=zeros(2*9*9,1);

for i=1:9
    % Left
    tmp=Ctrl_input;
    tmp(i)=tmp(i)-epsilon;
    Pert_Ctrl( 1+2*(i-1)*9:(2*i-1)*9 ) = tmp;
    % Right
    tmp=Ctrl_input;
    tmp(i)=tmp(i)+epsilon;
    Pert_Ctrl( 1+(2*i-1)*9 :2*i*9 ) = tmp;
end






end

== matlab function simulink_app/Flight mode manager and commands generator/Commands generator/commnads_gen_logic/commands_generator ==
  data: flight_mode input size=1; Xe input size=[3,1]; V_yaw input size=[3,1]; Euler input size=[3,1]; Loc_XY_sp output size=[2,1]; Alt_sp output size=1; Vel_yaw_xy_sp output size=[2,1]; Vel_yaw_z_sp output size=1; att_sp output size=[3,1]; omega_b_sp output size=[3,1]; K_alt output size=1; K_x output size=1; K_y output size=1; K_vx output size=1; K_vy output size=1; K_vz output size=1; K_phi output size=1; K_theta output size=1; K_yaw output size=1; K_p output size=1; K_q output size=1; K_r output size=1; Ix parameter size=1; Iy parameter size=1; Iz parameter size=1
function [Loc_XY_sp,Alt_sp,Vel_yaw_xy_sp,Vel_yaw_z_sp,att_sp,omega_b_sp , K_alt,K_x,K_y,K_vx,K_vy,K_vz,K_phi,K_theta,K_yaw,K_p,K_q,K_r]  =  commands_generator(flight_mode,Xe,V_yaw,Euler,Ix,Iy,Iz)
%% Generador de comandos (iniciales al menos) para cada fliht_mode



%% Pro precaucion, le damos la vuelta a la altura
Xe(3)=-Xe(3);

switch flight_mode
    case 0 % Off
        Loc_XY_sp       = [0,0]';
        Alt_sp          = 0; 
        Vel_yaw_xy_sp   = [0,0]';
        Vel_yaw_z_sp    = 0;
        att_sp          = [0,0,0]';
        omega_b_sp      = [0,0,0]';
        
        K_alt           = 0;
        K_x             = 0;
        K_y             = 0;
        K_vx            = 0;
        K_vy            = 0;
        K_vz            = 0;
        K_phi            = 0;
        K_theta            = 0;
        K_yaw           = 0;
        K_p            = 0;
        K_q            = 0;
        K_r            = 0;
    case 1 % Ready        
        Loc_XY_sp       = [0,0]';
        Alt_sp          = 0; 
        Vel_yaw_xy_sp   = [0,0]';
        Vel_yaw_z_sp    = 0;
        att_sp          = [0,0,0]';
        omega_b_sp      = [0,0,0]';

        K_alt           = 0;
        K_x             = 0;
        K_y             = 0;
        K_vx            = 0;
        K_vy            = 0;
        K_vz            = 0;
        K_phi           = 0;
        K_theta         = 0;
        K_yaw           = 0;

        K_p            = 0;
        K_q            = 0;
        K_r            = 0;
    case 2 % Take off
        Loc_XY_sp       = [0,0]';
        Alt_sp          = 1; 
        Vel_yaw_xy_sp   = [0,0]';
        Vel_yaw_z_sp    = 0;
        att_sp          = [0,0,Euler(3)]';
        omega_b_sp      = [0,0,0]';

        K_alt           = 1;
        K_x             = 0;
        K_y             = 0;
        K_vx            = 0;
        K_vy            = 0;
        K_vz            = 0;
        K_phi           = 0;
        K_theta        = 0;
        K_yaw           = 0;

        K_p            = 0;
        K_q            = 0;
        K_r            = 0;
    case 3 % Full_auto
        Loc_XY_sp       = [Xe(1),Xe(2)]';
        Alt_sp          = Xe(3); 
        Vel_yaw_xy_sp   = [0,0]';
        Vel_yaw_z_sp    = 0;
        att_sp          = [0,0,Euler(3)]';
        omega_b_sp      = [0,0,0]';

        K_alt           = 1;
        K_x             = 1;
        K_y             = 1;
        K_vx            = 0;
        K_vy            = 0;
        K_vz            = 0;
        K_phi            = 0;
        K_theta            = 0;
        K_yaw           = pi/180*(90);
        K_p            = 0;
        K_q            = 0;
        K_r            = 0;
    case 4 % Vel_height_auto
        Loc_XY_sp       = [0,0]';
        Alt_sp          = Xe(3); 
        Vel_yaw_xy_sp   = [0,0]';
        Vel_yaw_z_sp    = 0;
        att_sp          = [0,0,Euler(3)]';
        omega_b_sp      = [0,0,0]';

        K_alt           = 1;
        K_x             = 0;
        K_y             = 0;
        K_vx            = 1;
        K_vy            = 1;
        K_vz            = 0;
        K_phi            = 0;
        K_theta            = 0;
        K_yaw           = pi/180*(90);
        K_p            = 0;
        K_q            = 0;
        K_r            = 0;
    case 5 % Vel_auto
        Loc_XY_sp       = [0,0]';
        Alt_sp          = 0; 
        Vel_yaw_xy_sp   = [0,0]';
        Vel_yaw_z_sp    = 0;
        att_sp          = [0,0,Euler(3)]';
        omega_b_sp      = [0,0,0]';

        K_alt           = 0;
        K_x             = 0;
        K_y             = 0;
        K_vx            = 1;
        K_vy            = 1;
        K_vz            = 1;
        K_phi           = 0;
        K_theta         = 0;
        K_yaw           = pi/180*(90);
        K_p            = 0;
        K_q            = 0;
        K_r            = 0;
    case 6 % Stab
        Loc_XY_sp       = [0,0]';
        Alt_sp          = 0; 
        Vel_yaw_xy_sp   = [0,0]';
        Vel_yaw_z_sp    = 0;
        att_sp          = [0,0,Euler(3)]';
        omega_b_sp      = [0,0,0]';

        K_alt           = 0;
        K_x             = 0;
        K_y             = 0;
        K_vx            = 0;
        K_vy            = 0;
        K_vz            = 1;
        K_phi           = pi/180*10;
        K_theta         = pi/180*10;
        K_yaw           = pi/180*(90);
        K_p            = 0;
        K_q            = 0;
        K_r            = 0;
    case 7 % Man_ctrl
        Loc_XY_sp       = [0,0]';
        Alt_sp          = 0; 
        Vel_yaw_xy_sp   = [0,0]';
        Vel_yaw_z_sp    = 0;
        att_sp          = [0,0,0]';
        omega_b_sp      = [0,0,0]';

        K_alt           = 0;
        K_x             = 0;
        K_y             = 0;
        K_vx            = 0;
        K_vy            = 0;
        K_vz            = 1;
        K_phi           = 0;
        K_theta         = 0;
        K_yaw           = 0;
        K_p            = pi/180*(2);
        K_q            = pi/180*(2);
        K_r            = pi/180*(2);
    case 8 % Home
        Loc_XY_sp       = [0,0]';
        Alt_sp          = 0.5; 
        Vel_yaw_xy_sp   = [0,0]';
        Vel_yaw_z_sp    = 0;
        att_sp          = [0,0,Euler(3)]';
        omega_b_sp      = [0,0,0]';

        K_alt           = 0;
        K_x             = 0;
        K_y             = 0;
        K_vx            = 0;
        K_vy            = 0;
        K_vz            = 0;
        K_phi            = 0;
        K_theta            = 0;
        K_yaw           = 0;
        K_p            = 0;
        K_q            = 0;
        K_r            = 0;
    case 9 % Land
        Loc_XY_sp       = [Xe(1),Xe(2)]';
        Alt_sp          = 0; 
        Vel_yaw_xy_sp   = [0,0]';
        Vel_yaw_z_sp    = 0;
        att_sp          = [0,0,Euler(3)]';
        omega_b_sp      = [0,0,0]';

        K_alt           = 0;
        K_x             = 0;
        K_y             = 0;
        K_vx            = 0;
        K_vy            = 0;
        K_vz            = 0;
        K_phi            = 0;
        K_theta            = 0;
        K_yaw           = 0;
        K_p            = 0;
        K_q            = 0;
        K_r            = 0;
    otherwise
        Loc_XY_sp       = [0,0]';
        Alt_sp          = 0; 
        Vel_yaw_xy_sp   = [0,0]';
        Vel_yaw_z_sp    = 0;
        att_sp          = [0,0,Euler(3)]';
        omega_b_sp      = [0,0,0]';

        K_alt           = 0;
        K_x             = 0;
        K_y             = 0;
        K_vx            = 0;
        K_vy            = 0;
        K_vz            = 0;
        K_phi            = 0;
        K_theta            = 0;
        K_yaw           = 0;
        K_p            = 0;
        K_q            = 0;
        K_r            = 0;
end

== matlab function simulink_app/Flight mode manager and commands generator/Flight manager/Parameters_based_decision_making ==
  data: flight_mode_out output size=1; flight_mode input size=1; pdop input size=1; vdop input size=1; num_sats input size=1; Alt input size=1; Volt input size=1; Accs input size=[3,1]
function flight_mode_out     =  Params_decision_making(flight_mode,pdop,vdop,num_sats,Alt,Volt,Accs)

% si esta en landing y recive una aceleracion vertical de <-5m/s^2( Hacia
% arriba), pasar a modo OFF

% If ready from off blue LED
flight_mode_out = flight_mode;
 switch flight_mode % Being in this FM
        case 0 % Off
           
        case 1 % Ready
         
        case 2 % Take off
           
        case 3 % Full_auto
           
        case 4 % Vel_height_auto
           
        case 5 % Vel_auto
           
        case 6 % Stab
           
        case 7 % Man_ctrl
            
        case 8 % Home
            
        case 9 % Land
          
        otherwise
            flight_mode_out = flight_mode;
 end

== matlab function simulink_app/Flight mode manager and commands generator/Flight manager/flight_mode_manager ==
  data: flight_mode_reqest input size=1; Safety_stab_switch input size=1; flight_mode_out output size=1; p_dop input size=1; num_sats input size=1; Xe input size=[3,1]; Vyaw input size=[3,1]; Euler input size=[3,1]; Volt input size=1; flight_mode input size=1; NOT_allowed_sign output size=1
function [flight_mode_out,NOT_allowed_sign]   =  flight_mode_manager(flight_mode_reqest,Safety_stab_switch,p_dop,num_sats,Xe,Vyaw,Euler,Volt,flight_mode)
% Include here not allowed transitions of flight modes!!

%% monitor stab switch
if Safety_stab_switch==1
    flight_mode_reqest=6;
end

%% CHANGE ALTITUDE FOR WORKING ONLY WITH POSITIVE VALUES
Xe(3)=-Xe(3);


%% By default:
flight_mode_out = flight_mode; % Unless allowed change
NOT_allowed_sign = 0;

%% Allowed transitions logic
if flight_mode_reqest~=flight_mode
    switch flight_mode % Being in this FM
        case 0 % Off
            if flight_mode_reqest==1 && (num_sats>=4 && p_dop<2.5 && Volt > 14.0 && abs(Euler(1))<0.1 && abs(Euler(2))<0.1 )
                flight_mode_out = flight_mode_reqest;
            end
        case 1 % Ready
            if flight_mode_reqest==0
                flight_mode_out = flight_mode_reqest;
            end
            if flight_mode_reqest==2 && (num_sats>=4 && p_dop<2.5 && Volt > 14.0 && abs(Euler(1))<0.1 && abs(Euler(2))<0.1 ) % Add take off configuration
                flight_mode_out = flight_mode_reqest;
            end
        case 2 % Take off
            if (flight_mode_reqest==6 || flight_mode_reqest==7 || flight_mode_reqest==8 || flight_mode_reqest==9)
                flight_mode_out = flight_mode_reqest;
            end
            if (flight_mode_reqest==3 || flight_mode_reqest==4 || flight_mode_reqest==5) && (num_sats>=4 && p_dop<2.5 && abs(Euler(1))<0.1 && abs(Euler(2))<0.1 && Xe(3)>0.3 )
                flight_mode_out = flight_mode_reqest;
            end
            
        case 3 % Full_auto
            if (flight_mode_reqest==6 || flight_mode_reqest==7 || flight_mode_reqest==8 || flight_mode_reqest==9)
                flight_mode_out = flight_mode_reqest;
            end
            if ( flight_mode_reqest==4 || flight_mode_reqest==5) && (num_sats>=4 && p_dop<2.5 && abs(Euler(1))<0.1 && abs(Euler(2))<0.1 && Xe(3)>0.3 )
                flight_mode_out = flight_mode_reqest;
            end
        case 4 % Vel_height_auto
            if (flight_mode_reqest==6 || flight_mode_reqest==7 || flight_mode_reqest==8 || flight_mode_reqest==9)
                flight_mode_out = flight_mode_reqest;
            end
            if (flight_mode_reqest==3 || flight_mode_reqest==5) && (num_sats>=4 && p_dop<2.5 && abs(Euler(1))<0.1 && abs(Euler(2))<0.1 && Xe(3)>0.3 )
                flight_mode_out = flight_mode_reqest;
            end
        case 5 % Vel_auto
            if (flight_mode_reqest==6 || flight_mode_reqest==7 || flight_mode_reqest==8 || flight_mode_reqest==9)
                flight_mode_out = flight_mode_reqest;
            end
            if (flight_mode_reqest==3 || flight_mode_reqest==4 ) && (num_sats>=4 && p_dop<2.5 && abs(Euler(1))<0.1 && abs(Euler(2))<0.1 && Xe(3)>0.3 )
                flight_mode_out = flight_mode_reqest;
            end
        case 6 % Stab
            if ( flight_mode_reqest==7 || flight_mode_reqest==8 || flight_mode_reqest==9)
                flight_mode_out = flight_mode_reqest;
            end
            if (flight_mode_reqest==3 || flight_mode_reqest==4 || flight_mode_reqest==5) && (num_sats>=4 && p_dop<2.5 && abs(Euler(1))<0.1 && abs(Euler(2))<0.1 && Xe(3)>0.3 )
                flight_mode_out = flight_mode_reqest;
            end
        case 7 % Man_ctrl
            if (flight_mode_reqest==6 || flight_mode_reqest==8 || flight_mode_reqest==9)
                flight_mode_out = flight_mode_reqest;
            end
            if (flight_mode_reqest==3 || flight_mode_reqest==4 || flight_mode_reqest==5) && (num_sats>=4 && p_dop<2.5 && abs(Euler(1))<0.1 && abs(Euler(2))<0.1 && Xe(3)>0.3 )
                flight_mode_out = flight_mode_reqest;
            end
        case 8 % Home
            if (flight_mode_reqest==6 || flight_mode_reqest==7 || flight_mode_reqest==9)
                flight_mode_out = flight_mode_reqest;
            end
            if (flight_mode_reqest==3 || flight_mode_reqest==4 || flight_mode_reqest==5) && (num_sats>=4 && p_dop<2.5 && abs(Euler(1))<0.1 && abs(Euler(2))<0.1 && Xe(3)>0.3 )
                flight_mode_out = flight_mode_reqest;
            end
        case 9 % Land
            if (flight_mode_reqest==1 || flight_mode_reqest==2)
                flight_mode_out = flight_mode_reqest;
            end
        otherwise
            flight_mode_out = flight_mode; % Unless allowed change
            
    end
    

end

% If not allowed change:
if flight_mode_reqest~=flight_mode_out
    NOT_allowed_sign = 1; % Make anything
end

== matlab function simulink_app/Px4_to_simulink input interface/MATLAB Function ==
  data: T_yaw output size=[3,3]; yaw input size=1
function T_yaw = Yaw_rotate(yaw)


T_yaw=[cos(yaw),    sin(yaw),   0;
        -sin(yaw),  cos(yaw),   0;
        0,      0,              1];
